simulink model "system_simulation"  (R2020a)
settings: Solver=VariableStepAuto  StartTime=0.0  StopTime=1000  RelTol=1e-3
InitFcn:
  | LAB2
values from neighbouring files (symbols this model uses):
  A = [-0.342 0 0.0318; 0 -0.0716 0.0318; 0.0204 0.0204 -0.0423]    [LAB2.m]
  B = [0.159 0; 0 0.159; 0 0]    [LAB2.m]
  C = [1 0 0; 0 1 0]    [LAB2.m]
settings Model: Creator=paulogil  LastModifiedBy=joaom
settings OptimizationCC: LifeSpan=inf
settings DebuggingCC: SFExecutionAtInitializationDiag=none  ArithmeticOperatorsInVariantConditions=warning
settings SFSimCC: CustomCodeUndefinedFunction=UseInterfaceOnly
settings CodeAppCC: StateflowObjectComments=on

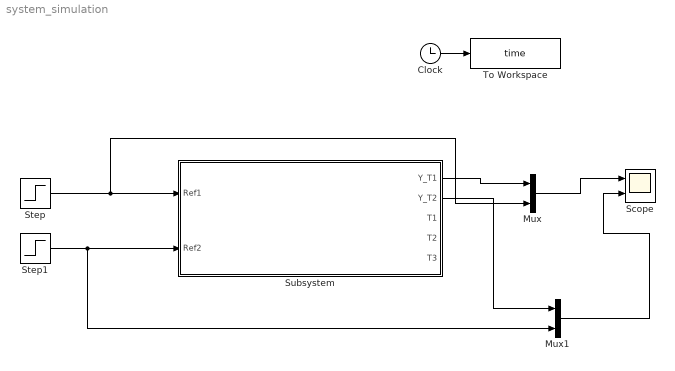
== system system_simulation ==
  Clock : Clock
  Mux : Mux  Inputs=2
  Mux1 : Mux  Inputs=2
  Scope : Scope  NumInputPorts=2
  Step : Step  Time=0  SampleTime=0
  Step1 : Step  SampleTime=0
  Subsystem : Subsystem
  To Workspace : ToWorkspace  VariableName=time  SaveFormat=Timeseries  SampleTime=-1
  wires:
  Clock/1 -> To Workspace/1
  Step/1 -> Mux/2, Subsystem/1(Ref1)
  Step1/1 -> Mux1/2, Subsystem/2(Ref2)
  Subsystem/1(Y_T1) -> Mux/1
  Mux/1 -> Scope/1
  Mux1/1 -> Scope/2
  Subsystem/2(Y_T2) -> Mux1/1

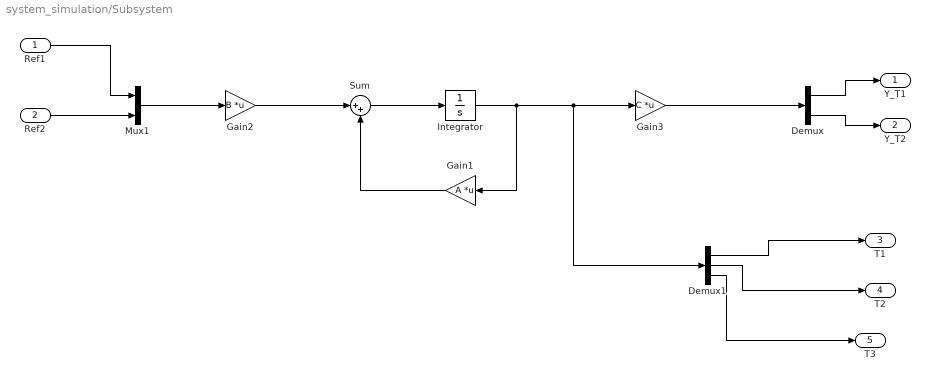
== system system_simulation/Subsystem ==
  Ref1 : Inport
  Ref2 : Inport  Port=2
  Demux : Demux  Outputs=2
  Demux1 : Demux  Outputs=3
  Gain1 : Gain  Gain=A  Multiplication=Matrix(K*u)
  Gain2 : Gain  Gain=B  Multiplication=Matrix(K*u)
  Gain3 : Gain  Gain=C  Multiplication=Matrix(K*u)
  Integrator : Integrator
  Mux1 : Mux  Inputs=2
  Sum : Sum  Inputs=|++
  Y_T1 : Outport
  Y_T2 : Outport  Port=2
  T1 : Outport  Port=3
  T2 : Outport  Port=4
  T3 : Outport  Port=5
  wires:
  Gain2/1 -> Sum/1
  Ref1/1 -> Mux1/1
  Gain1/1 -> Sum/2
  Integrator/1 -> Demux1/1, Gain3/1, Gain1/1
  Sum/1 -> Integrator/1
  Mux1/1 -> Gain2/1
  Ref2/1 -> Mux1/2
  Gain3/1 -> Demux/1
  Demux/1 -> Y_T1/1
  Demux/2 -> Y_T2/1
  Demux1/1 -> T1/1
  Demux1/2 -> T2/1
  Demux1/3 -> T3/1
